simulink model "fuzzy_controller"  (R2024a)
settings: Solver=FixedStepAuto  StartTime=0.0  StopTime=20  FixedStep=0.01  RelTol=1e-3
libraries: fuzblock x1
settings Model: Creator=VKIST  LastModifiedBy=TRUONG GIANG
settings DebuggingCC: UnconnectedInputMsg=warning  UnconnectedOutputMsg=warning  UnconnectedLineMsg=warning
settings ModelReferenceCC: EnableRefExpFcnMdlSchedulingChecks=on
settings RTWCC: GPUComputeCapability=3.5  DLArmComputeVersion=19.05

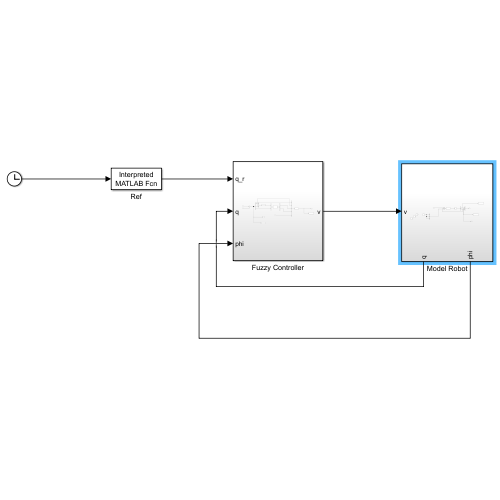
[thumbnail: Simulink's stored preview of the top-level diagram]
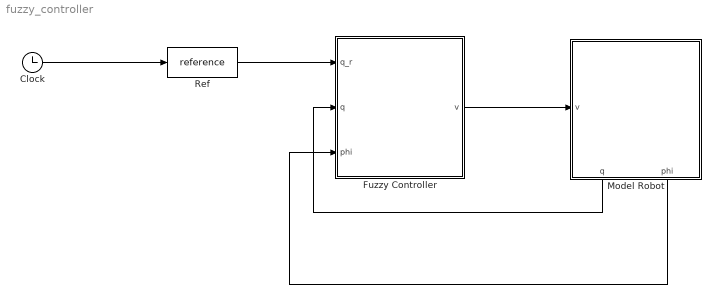
== system fuzzy_controller ==
  Clock : Clock
      settings: Decimation=20
  Fuzzy Controller : Subsystem
  Model Robot : Subsystem
      settings: PortSchema="{\"entries\":[{\"content\":{\"sides\":[{\"content\":{\"connectorIds\":[\"In1\"]},\"type\":\"ConnectorPlacement.EquallySpacedRectSide\",\"uuid\":\"b3721482-5ff4-4937-a09e-80084b1ea56b\"},{\"content\":{\"connectorIds\":[],\"side\":\"RIGHT\"},\"type\":\"ConnectorPlacement.EquallySpacedRectSide\",\"uuid\":\"d3d37232-6b83-4f62-8c12-a0abf7cc0899\"},{\"content\":{\"connectorIds\":[],\"side\":\"TOP\"},\"type\":\"ConnectorPlacement.EquallySpacedRectSide\",\"uuid\":\"c74b4e0a-6064-492f-9200-196cab4f263e\"},{\"content\":{\"connectorIds\":[\"Out1\",\"Out2\"],\"side\":\"BOTTOM\"},\"type\":\"ConnectorPlacement.EquallySpacedRectSide\",\"uuid\":\"5d2d1d78-4924-4e2c-8792-a7212ffd26ec\"}]},\"type\":\"ConnectorPlacement.EquallySpacedConnector\",\"uuid\":\"27b4ec6a-90c7-4f9f-8ee2-7c9cc7945c61\"}],\"packageUris\":[\"http://schema.mathworks.com/mf0/Connector/R2020b\"],\"version\":\"1.0\"}"
  Ref : MATLABFcn  MATLABFcn=reference  OutputDimensions=3
  wires:
  Ref/1 -> Fuzzy Controller/1(q_r)
  Clock/1 -> Ref/1
  Fuzzy Controller/1(v) -> Model Robot/1(v)
  Model Robot/1(q) -> Fuzzy Controller/2(q)
  Model Robot/2(phi) -> Fuzzy Controller/3(phi)

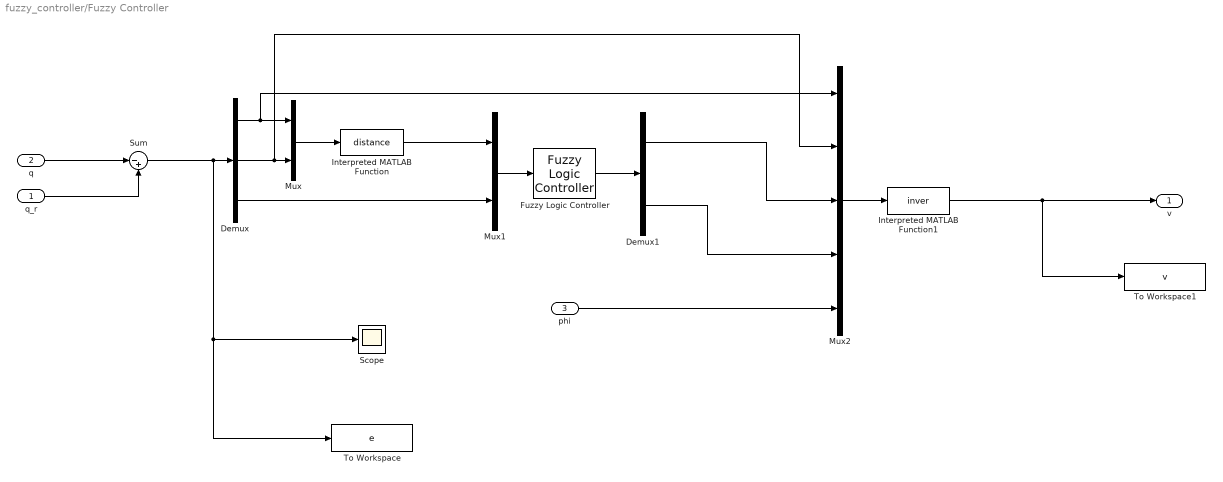
== system fuzzy_controller/Fuzzy Controller ==
  q_r : Inport
  q : Inport  Port=2
  phi : Inport  Port=3
  Demux : Demux  Outputs=3
  Demux1 : Demux  Outputs=2
  Fuzzy Logic Controller : fuzblock/Fuzzy Logic  Controller  FIS='fuzzy3.fis'  OutputSampleNumber=101  DataType=double  FuzzifiedInputs=off  RuleFiringStrengths=off  RuleOutputs=off  AggregatedOutputs=off  SimulateUsing=Interpreted execution  OutOfRangeInputValueMessage=warning  NoRuleFiredMessage=warning  EmptyOutputFuzzySetMessage=warning
  Interpreted MATLAB Function : MATLABFcn  MATLABFcn=distance  OutputDimensions=1
  Interpreted MATLAB Function1 : MATLABFcn  MATLABFcn=inver  OutputDimensions=3
  Mux : Mux  Inputs=2
  Mux1 : Mux  Inputs=2
  Mux2 : Mux  Inputs=5
  Scope : Scope
  Sum : Sum  Inputs=|-+
  To Workspace : ToWorkspace  VariableName=e  SampleTime=-1
  To Workspace1 : ToWorkspace  VariableName=v  SampleTime=-1
  v : Outport
  wires:
  q/1 -> Sum/1
  q_r/1 -> Sum/2
  Sum/1 -> Scope/1, To Workspace/1, Demux/1
  Demux/2 -> Mux2/2, Mux/2
  Demux/1 -> Mux/1, Mux2/1
  Mux/1 -> Interpreted MATLAB Function/1
  Mux1/1 -> Fuzzy Logic Controller/1
  Interpreted MATLAB Function/1 -> Mux1/1
  Demux/3 -> Mux1/2
  Fuzzy Logic Controller/1 -> Demux1/1
  Mux2/1 -> Interpreted MATLAB Function1/1
  Demux1/1 -> Mux2/3
  Demux1/2 -> Mux2/4
  Interpreted MATLAB Function1/1 -> v/1, To Workspace1/1
  phi/1 -> Mux2/5

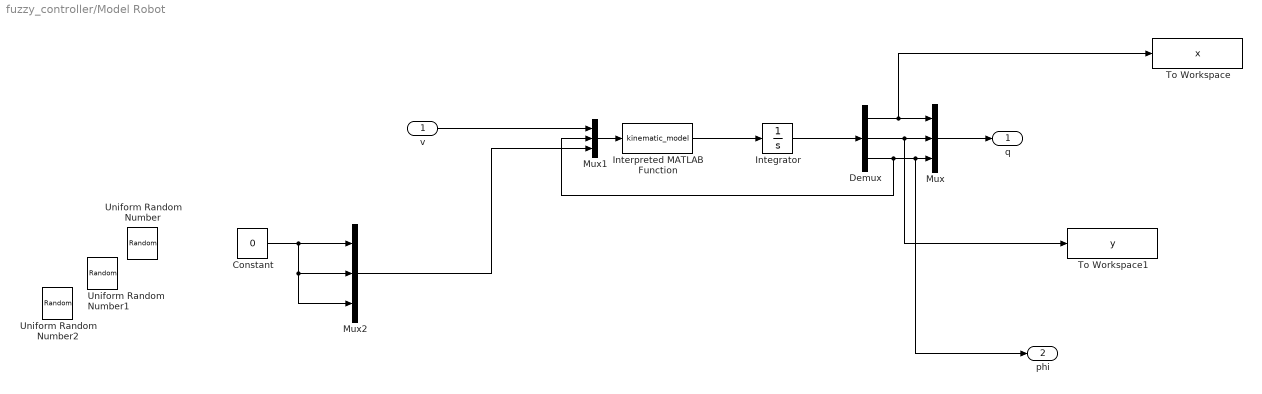
== system fuzzy_controller/Model Robot ==
  v : Inport
  Constant : Constant  Value=0
  Demux : Demux  Outputs=3
  Integrator : Integrator
  Interpreted MATLAB Function : MATLABFcn  MATLABFcn=kinematic_model  OutputDimensions=3
  Mux : Mux  Inputs=3
  Mux1 : Mux  Inputs=3
  Mux2 : Mux  Inputs=3
  To Workspace : ToWorkspace  VariableName=x  SampleTime=-1
  To Workspace1 : ToWorkspace  VariableName=y  SampleTime=-1
  Uniform Random Number : UniformRandomNumber  SampleTime=0.1
  Uniform Random Number1 : UniformRandomNumber  SampleTime=0.1
  Uniform Random Number2 : UniformRandomNumber  SampleTime=0.1
  q : Outport
  phi : Outport  Port=2
  wires:
  Interpreted MATLAB Function/1 -> Integrator/1
  Integrator/1 -> Demux/1
  Demux/2 -> To Workspace1/1, Mux/2
  Demux/3 -> Mux1/2, phi/1, Mux/3
  Demux/1 -> To Workspace/1, Mux/1
  Mux/1 -> q/1
  Mux1/1 -> Interpreted MATLAB Function/1
  v/1 -> Mux1/1
  Mux2/1 -> Mux1/3
  Constant/1 -> Mux2/2, Mux2/3, Mux2/1
